simulink model "MIL_model"  (R2024b)
settings: Solver=ode4  StartTime=0.0  StopTime=T_stop  FixedStep=0.1  RelTol=1e-3
PreLoadFcn:
  | run(fullfile(fileparts(which('MIL_model')), '..' , 'scripts', 'init_MIL_model.m'));
undefined symbols (not defined in the file): dt, SoC_init, T_cool_init, V_RC1_init, V_RC2_init
libraries: simulink x1
settings Model: DataDictionary=buses.sldd  Creator=rayen  LastModifiedBy=rayen
settings DebuggingCC: AlgebraicLoopMsg=error

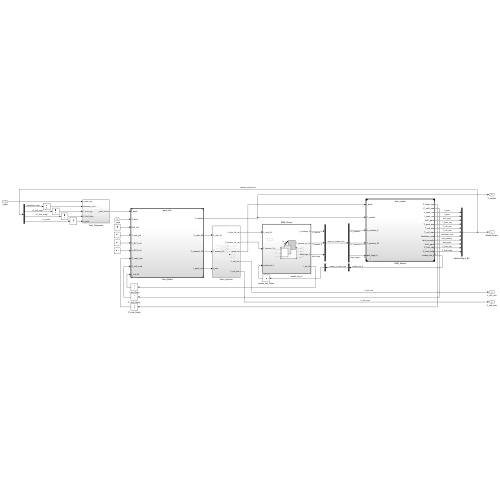
[thumbnail: Simulink's stored preview of the top-level diagram]
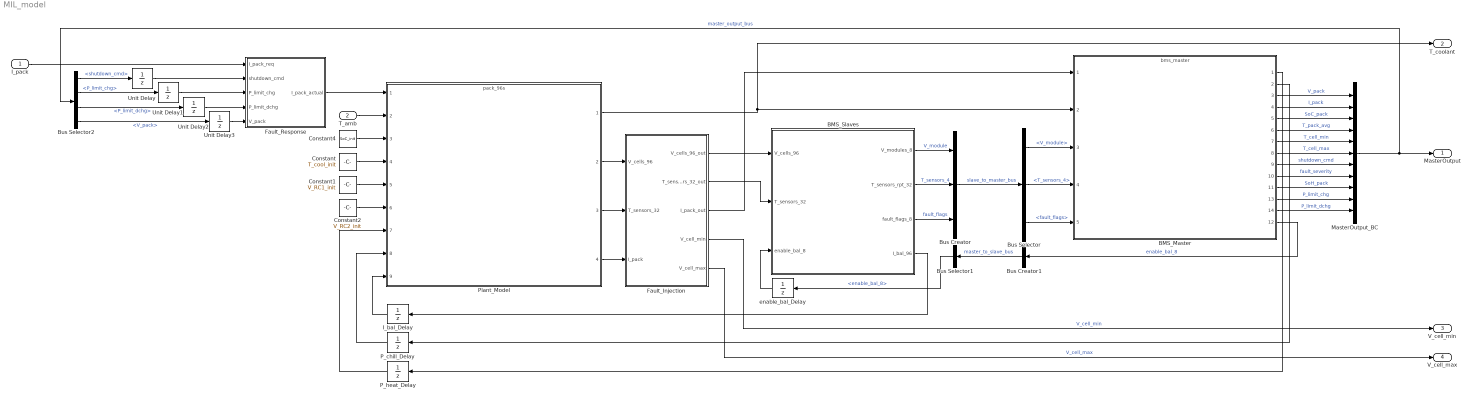
== system MIL_model ==
  I_pack : Inport  OutDataTypeStr=double
  T_amb : Inport  Port=2  OutDataTypeStr=double
  BMS_Master : ModelReference  ModelNameDialog=bms_master  ModelReferenceVersion=1.183
      settings: PortSchema="{\"entries\":[{\"content\":{\"sides\":[{\"content\":{\"connectorIds\":[\"In1\",\"In2\",\"In3\",\"In4\",\"In5\"]},\"type\":\"ConnectorPlacement.EquallySpacedRectSide\",\"uuid\":\"8066489d-2b28-420f-9202-9cd6ff178a29\"},{\"content\":{\"connectorIds\":[\"Out1\",\"Out2\",\"Out3\",\"Out4\",\"Out5\",\"Out6\",\"Out7\",\"Out8\",\"Out9\",\"Out10\",\"Out11\",\"Out13\",\"Out14\",\"Out12\"],\"side\":\"RIGHT\"},\"type\":\"ConnectorPlacement.EquallySpacedRectSide\",\"uuid\":\"b076ecb5-2558-4b32-94db-f7a524b49e8a\"},{\"content\":{\"side\":\"TOP\"},\"type\":\"ConnectorPlacement.EquallySpacedRectSide\",\"uuid\":\"5bce71a0-8ae7-4a96-a6b6-c7adac2010e7\"}]},\"type\":\"ConnectorPlacement.EquallySpacedConnector\",\"uuid\":\"27e9bc73-c1a9-451e-b2df-2718d4e67b4c\"}],\"packageUris\":[\"http://schema.mathworks.com/mf0/Connector/R2020b\"],\"version\":\"1.0\"}"
  BMS_Slaves : Subsystem  TreatAsAtomicUnit=on
  Bus Creator : BusCreator  Inputs=3
  Bus Creator1 : BusCreator  Inputs=1
  Bus Selector : BusSelector  OutputSignals=V_module,T_sensors_4,fault_flags
  Bus Selector1 : BusSelector  OutputSignals=enable_bal_8
  Bus Selector2 : BusSelector  OutputSignals=shutdown_cmd,P_limit_chg,P_limit_dchg,V_pack
  Constant : Constant  Value=T_cool_init
  Constant1 : Constant  Value=V_RC1_init
  Constant2 : Constant  Value=V_RC2_init
  Constant4 : Constant  Value=SoC_init
  Fault_Injection : Subsystem
  Fault_Response : Subsystem
  I_bal_Delay : UnitDelay  InitialCondition=zeros(12,8)  SampleTime=dt  HasFrameUpgradeWarning=on
  MasterOutput_BC : BusCreator  Inputs=11
  P_chill_Delay : UnitDelay  SampleTime=dt  HasFrameUpgradeWarning=on
  P_heat_Delay : UnitDelay  SampleTime=dt  HasFrameUpgradeWarning=on
  Plant_Model : ModelReference  ModelNameDialog=pack_96s.slx  SimulationMode=Normal  ModelReferenceVersion=1.64
  Unit Delay : UnitDelay  SampleTime=dt  HasFrameUpgradeWarning=on
  Unit Delay1 : UnitDelay  InitialCondition=96*4.2*150  SampleTime=dt  HasFrameUpgradeWarning=on
  Unit Delay2 : UnitDelay  InitialCondition=96*2.5*405  SampleTime=dt  HasFrameUpgradeWarning=on
  Unit Delay3 : UnitDelay  InitialCondition=96*3.7  SampleTime=dt  HasFrameUpgradeWarning=on
  enable_bal_Delay : UnitDelay  InitialCondition=zeros(1,8)  SampleTime=dt  HasFrameUpgradeWarning=on
  MasterOutput : Outport
  T_coolant : Outport  Port=2
  V_cell_min : Outport  Port=3
  V_cell_max : Outport  Port=4
  wires:
  T_amb/1 -> Plant_Model/2
  Constant/1 -> Plant_Model/4
  Constant2/1 -> Plant_Model/6
  Constant4/1 -> Plant_Model/3
  Constant1/1 -> Plant_Model/5
  P_heat_Delay/1 -> Plant_Model/7
  Plant_Model/1 -> T_coolant/1, BMS_Master/2
  enable_bal_Delay/1 -> BMS_Slaves/3(enable_bal_8)
  BMS_Slaves/4(I_bal_96) -> I_bal_Delay/1
  BMS_Master/3 -> MasterOutput_BC/1  "V_pack"
  BMS_Master/1 -> P_heat_Delay/1
  BMS_Master/4 -> MasterOutput_BC/2  "I_pack"
  BMS_Master/2 -> P_chill_Delay/1
  BMS_Master/11 -> MasterOutput_BC/9  "SoH_pack"
  BMS_Master/9 -> MasterOutput_BC/7  "shutdown_cmd"
  BMS_Master/7 -> MasterOutput_BC/5  "T_cell_min"
  BMS_Master/5 -> MasterOutput_BC/3  "SoC_pack"
  BMS_Master/10 -> MasterOutput_BC/8  "fault_severity"
  BMS_Master/8 -> MasterOutput_BC/6  "T_cell_max"
  BMS_Master/6 -> MasterOutput_BC/4  "T_pack_avg"
  I_bal_Delay/1 -> Plant_Model/9
  MasterOutput_BC/1 -> MasterOutput/1, Bus Selector2/1  "master_output_bus"
  P_chill_Delay/1 -> Plant_Model/8
  BMS_Slaves/3(fault_flags_8) -> Bus Creator/3  "fault_flags"
  BMS_Slaves/2(T_sensors_rpt_32) -> Bus Creator/2  "T_sensors_4"
  BMS_Slaves/1(V_modules_8) -> Bus Creator/1  "V_module"
  Bus Creator/1 -> Bus Selector/1  "slave_to_master_bus"
  BMS_Master/12 -> Bus Creator1/1  "enable_bal_8"
  Bus Creator1/1 -> Bus Selector1/1  "master_to_slave_bus"
  Bus Selector1/1 -> enable_bal_Delay/1  "<enable_bal_8>"
  Fault_Response/1(I_pack_actual) -> Plant_Model/1
  I_pack/1 -> Fault_Response/1(I_pack_req)
  BMS_Master/13 -> MasterOutput_BC/10  "P_limit_chg"
  BMS_Master/14 -> MasterOutput_BC/11  "P_limit_dchg"
  Bus Selector/1 -> BMS_Master/3  "<V_module>"
  Bus Selector/2 -> BMS_Master/4  "<T_sensors_4>"
  Bus Selector/3 -> BMS_Master/5  "<fault_flags>"
  Unit Delay2/1 -> Fault_Response/4(P_limit_dchg)
  Bus Selector2/2 -> Unit Delay1/1  "<P_limit_chg>"
  Unit Delay3/1 -> Fault_Response/5(V_pack)
  Bus Selector2/4 -> Unit Delay3/1  "<V_pack>"
  Unit Delay1/1 -> Fault_Response/3(P_limit_chg)
  Unit Delay/1 -> Fault_Response/2(shutdown_cmd)
  Bus Selector2/1 -> Unit Delay/1  "<shutdown_cmd>"
  Bus Selector2/3 -> Unit Delay2/1  "<P_limit_dchg>"
  Plant_Model/2 -> Fault_Injection/1(V_cells_96)
  Plant_Model/3 -> Fault_Injection/2(T_sensors_32)
  Plant_Model/4 -> Fault_Injection/3(I_pack)
  Fault_Injection/1(V_cells_96_out) -> BMS_Slaves/1(V_cells_96)
  Fault_Injection/2(T_sensors_32_out) -> BMS_Slaves/2(T_sensors_32)
  Fault_Injection/3(I_pack_out) -> BMS_Master/1
  Fault_Injection/5(V_cell_max) -> V_cell_max/1  "V_cell_max"
  Fault_Injection/4(V_cell_min) -> V_cell_min/1  "V_cell_min"

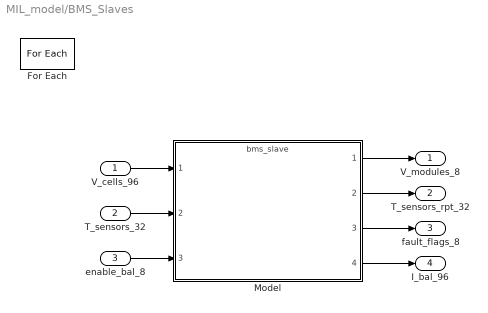
== system MIL_model/BMS_Slaves ==
  V_cells_96 : Inport  Partition=on  PartitionDimension=1  PartitionWidth=12  PartitionOffset=0
  T_sensors_32 : Inport  Port=2  Partition=on  PartitionDimension=1  PartitionWidth=4  PartitionOffset=0
  enable_bal_8 : Inport  Port=3  Partition=on  PartitionDimension=1  PartitionWidth=1  PartitionOffset=0
  For Each : ForEach  DisableCoverage=on
  Model : ModelReference  ModelNameDialog=bms_slave.slx  ModelReferenceVersion=1.55
  V_modules_8 : Outport  ConcatenationDimension=1
  T_sensors_rpt_32 : Outport  Port=2  ConcatenationDimension=1
  fault_flags_8 : Outport  Port=3  ConcatenationDimension=1
  I_bal_96 : Outport  Port=4  ConcatenationDimension=2
  wires:
  enable_bal_8/1 -> Model/3
  T_sensors_32/1 -> Model/2
  V_cells_96/1 -> Model/1
  Model/1 -> V_modules_8/1
  Model/2 -> T_sensors_rpt_32/1
  Model/3 -> fault_flags_8/1
  Model/4 -> I_bal_96/1

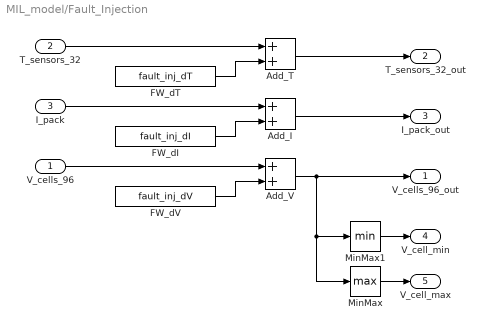
== system MIL_model/Fault_Injection ==
  V_cells_96 : Inport
  T_sensors_32 : Inport  Port=2
  I_pack : Inport  Port=3
  Add_I : Sum
  Add_T : Sum
  Add_V : Sum
  FW_dI : FromWorkspace  VariableName=fault_inj_dI  Interpolate=off  OutputAfterFinalValue=Holding final value
  FW_dT : FromWorkspace  VariableName=fault_inj_dT  Interpolate=off  OutputAfterFinalValue=Holding final value
  FW_dV : FromWorkspace  VariableName=fault_inj_dV  Interpolate=off  OutputAfterFinalValue=Holding final value
  MinMax : MinMax  Function=max
  MinMax1 : MinMax
  V_cells_96_out : Outport
  T_sensors_32_out : Outport  Port=2
  I_pack_out : Outport  Port=3
  V_cell_min : Outport  Port=4
  V_cell_max : Outport  Port=5
  wires:
  V_cells_96/1 -> Add_V/1
  FW_dV/1 -> Add_V/2
  Add_V/1 -> V_cells_96_out/1, MinMax1/1, MinMax/1
  T_sensors_32/1 -> Add_T/1
  FW_dT/1 -> Add_T/2
  Add_T/1 -> T_sensors_32_out/1
  I_pack/1 -> Add_I/1
  FW_dI/1 -> Add_I/2
  Add_I/1 -> I_pack_out/1
  MinMax/1 -> V_cell_max/1
  MinMax1/1 -> V_cell_min/1

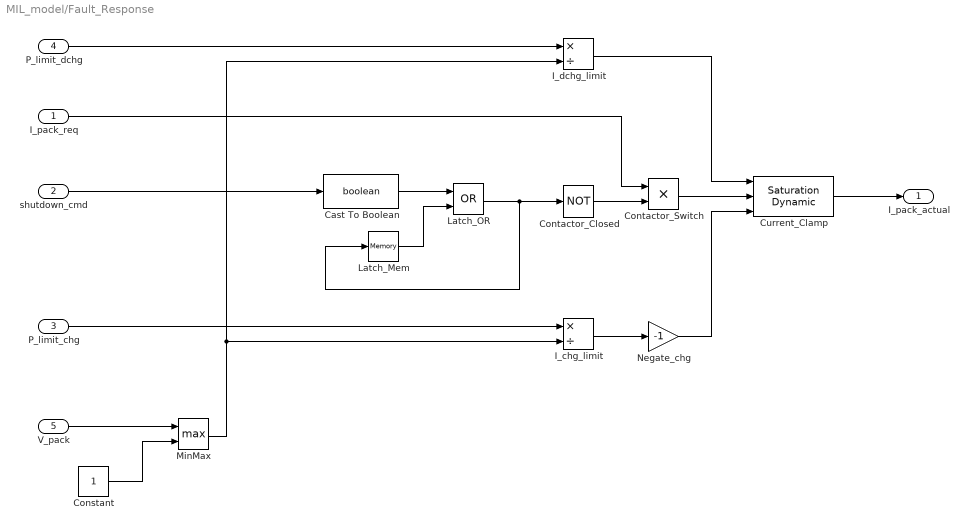
== system MIL_model/Fault_Response ==
  I_pack_req : Inport
  shutdown_cmd : Inport  Port=2
  P_limit_chg : Inport  Port=3
  P_limit_dchg : Inport  Port=4
  V_pack : Inport  Port=5
  Cast To Boolean : DataTypeConversion  OutDataTypeStr=boolean  SaturateOnIntegerOverflow=off  RndMeth=Floor
  Constant : Constant
  Contactor_Closed : Logic  Operator=NOT  AllPortsSameDT=off  OutDataTypeStr=boolean
  Contactor_Switch : Product
  Current_Clamp : simulink/Discontinuities/Saturation Dynamic  OutMin=[]  OutMax=[]  OutDataTypeStr=Inherit: Same as second input  OutDataType=fixdt(1, 16)  OutScaling=2^-10  DoSatur=off
  I_chg_limit : Product  Inputs=*/
  I_dchg_limit : Product  Inputs=*/
  Latch_Mem : Memory
  Latch_OR : Logic  Operator=OR  AllPortsSameDT=off  OutDataTypeStr=boolean
  MinMax : MinMax  Function=max  Inputs=2
  Negate_chg : Gain  Gain=-1
  I_pack_actual : Outport
  wires:
  Latch_Mem/1 -> Latch_OR/2
  Latch_OR/1 -> Latch_Mem/1, Contactor_Closed/1
  Contactor_Closed/1 -> Contactor_Switch/2
  I_pack_req/1 -> Contactor_Switch/1
  P_limit_chg/1 -> I_chg_limit/1
  V_pack/1 -> MinMax/1
  I_chg_limit/1 -> Negate_chg/1
  P_limit_dchg/1 -> I_dchg_limit/1
  Contactor_Switch/1 -> Current_Clamp/2
  I_dchg_limit/1 -> Current_Clamp/1
  Negate_chg/1 -> Current_Clamp/3
  Current_Clamp/1 -> I_pack_actual/1
  Constant/1 -> MinMax/2
  MinMax/1 -> I_chg_limit/2, I_dchg_limit/2
  Cast To Boolean/1 -> Latch_OR/1
  shutdown_cmd/1 -> Cast To Boolean/1
